simulink model "DC_Motor_Load"  (R2015a)
settings: Solver=ode45  StartTime=0.0  StopTime=10.0  RelTol=1e-3
values from neighbouring files (symbols this model uses):
  BL = B_roller + B_material    (= 0)    [dc_motor_show_data_last.m]    (also in dc_motor_show_data_last_pos.m)
  Bm = 0.0158    [dc_motor_show_data_last.m]    (also in dc_motor_show_data_last_pos.m = 0.00093)
  JL = J_roller + J_material    (= 0.000102958)    [dc_motor_show_data_last.m]    (also in dc_motor_show_data_last_pos.m)
  Jm = 0.00252    [dc_motor_show_data_last.m]    (also in dc_motor_show_data_last_pos.m = 5.26e-05)
  Kd = Kp*Td    (= 8.33268608414)    [ZIEGLER_NICHOLCUS_METHOD_tuning_pid.m]    (also in dc_motor_show_data.m = 0.0189; dc_motor_show_data_PID_range_errors_show.m = 0.09; dc_motor_show_data_PID_range_response.m = 0.09; dc_motor_show_data_PID_test_ST.m = 0.09)
  Ke = 0.1    [DC_MOTOR.m]    (also in ZIEGLER_NICHOLCUS_METHOD_tuning_pid.m = 0.57; dc_motor_show_data.m = 0.57; dc_motor_show_data_PID_range_errors_show.m; dc_motor_show_data_PID_range_response.m)
  Ki = Kp/Ti    (= 21.5184713376)    [ZIEGLER_NICHOLCUS_METHOD_tuning_pid.m]    (also in dc_motor_show_data.m = 39.9; dc_motor_show_data_PID_range_errors_show.m = 2.98; dc_motor_show_data_PID_range_response.m = 2.98; dc_motor_show_data_PID_test_ST.m = 2.98)
  Kp = 0.2*K_cr    (= 16.4)    [ZIEGLER_NICHOLCUS_METHOD_tuning_pid.m]    (also in dc_motor_show_data.m = 2.1398; dc_motor_show_data_PID_range_errors_show.m = 1.25; dc_motor_show_data_PID_range_response.m = 1.25; dc_motor_show_data_PID_test_ST.m = 1.25)
  Kt = 0.2    [DC_MOTOR.m]    (also in ZIEGLER_NICHOLCUS_METHOD_tuning_pid.m = 0.259; dc_motor_show_data.m = 0.259; dc_motor_show_data_PID_range_errors_show.m; dc_motor_show_data_PID_range_response.m)
  La = 0.143    [dc_motor_show_data_last.m]    (also in dc_motor_show_data_last_pos.m = 0.0006)
  Ra = 9.375    [dc_motor_show_data_last.m]    (also in dc_motor_show_data_last_pos.m)
  TL = 0.0017    [dc_motor_show_data_last.m]    (also in dc_motor_show_data_last_pos.m)
libraries: simulink x1
settings Model: Creator=Alfa maSR  LastModifiedBy=Alfa maSR

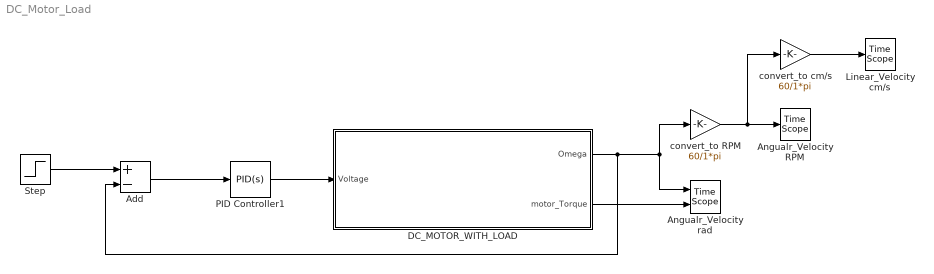
== system DC_Motor_Load ==
  Add : Sum  Inputs=+-
  Angualr_Velocity RPM : TimeScope  DefaultConfigurationName=spbscopes.TimeScopeBlockCfg
  Angualr_Velocity rad : TimeScope  DefaultConfigurationName=spbscopes.TimeScopeBlockCfg  NumInputPorts=2
  DC_MOTOR_WITH_LOAD : Subsystem
  Linear_Velocity cm/s : TimeScope  DefaultConfigurationName=spbscopes.TimeScopeBlockCfg
  PID Controller1 : simulink/Continuous/PID Controller  Controller=PID  TimeDomain=Continuous-time  SampleTime=-1  IntegratorMethod=Forward Euler  FilterMethod=Forward Euler  Form=Parallel  UseFilter=on  ControllerParametersSource=internal  P=Kp  I=Ki  D=Kd  N=100  InitialConditionSource=internal  InitialConditionForIntegrator=0  InitialConditionForFilter=0  ExternalReset=none  LimitOutput=off  UpperSaturationLimit=inf  LowerSaturationLimit=-inf  LinearizeAsGain=on  AntiWindupMode=none  Kb=1  TrackingMode=off  Kt=1  PParamMin=[]  PParamMax=[]  IParamMin=[]  IParamMax=[]  DParamMin=[]  DParamMax=[]  NParamMin=[]  NParamMax=[]  KbParamMin=[]  KbParamMax=[]  KtParamMin=[]  KtParamMax=[]  POutMin=[]  POutMax=[]  IOutMin=[]  IOutMax=[]  DOutMin=[]  DOutMax=[]  NOutMin=[]  NOutMax=[]  KbOutMin=[]  KbOutMax=[]  KtOutMin=[]  KtOutMax=[]  IntegratorOutMin=[]  IntegratorOutMax=[]  FilterOutMin=[]  FilterOutMax=[]  SumOutMin=[]  SumOutMax=[]  SumI1OutMin=[]  SumI1OutMax=[]  SumI2OutMin=[]  SumI2OutMax=[]  SumI3OutMin=[]  SumI3OutMax=[]  SumDOutMin=[]  SumDOutMax=[]  SaturationOutMin=[]  SaturationOutMax=[]  IntegratorContinuousStateAttributes=''  IntegratorStateMustResolveToSignalObject=off  IntegratorRTWStateStorageClass=Auto  FilterContinuousStateAttributes=''  FilterStateMustResolveToSignalObject=off  FilterRTWStateStorageClass=Auto  DifferentiatorICPrevScaledInput=0  DifferentiatorOutMin=[]  DifferentiatorOutMax=[]
  Step : Step  Time=0  SampleTime=0
  convert_to RPM : Gain  Gain=60/1*pi
  convert_to cm/s : Gain  Gain=60/1*pi
  wires:
  convert_to RPM/1 -> Angualr_Velocity RPM/1, convert_to cm/s/1
  convert_to cm/s/1 -> Linear_Velocity cm/s/1
  DC_MOTOR_WITH_LOAD/1(Omega) -> Add/2, convert_to RPM/1, Angualr_Velocity rad/1
  DC_MOTOR_WITH_LOAD/2(motor_Torque) -> Angualr_Velocity rad/2
  PID Controller1/1 -> DC_MOTOR_WITH_LOAD/1(Voltage)
  Add/1 -> PID Controller1/1
  Step/1 -> Add/1

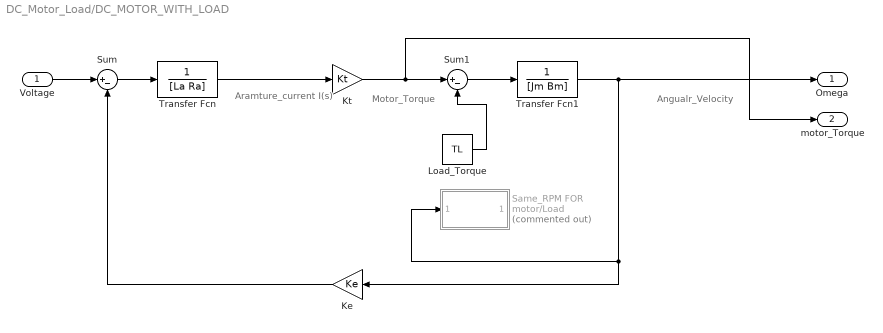
== system DC_Motor_Load/DC_MOTOR_WITH_LOAD ==
  note: Angualr_Velocity
  note: Motor_Torque
  note: Aramture_current
      |           I(s)
  Voltage : Inport
  Ke : Gain  Gain=Ke
  Kt : Gain  Gain=Kt
  Load_Torque : Constant  Value=TL
  Same_RPM FOR motor/Load : Subsystem  Commented=on
  Sum : Sum  Inputs=|+-
  Sum1 : Sum  Inputs=|+-
  Transfer Fcn : TransferFcn  Denominator=[La Ra]
  Transfer Fcn1 : TransferFcn  Denominator=[Jm Bm]
  Omega : Outport
  motor_Torque : Outport  Port=2
  wires:
  Ke/1 -> Sum/2
  Sum1/1 -> Transfer Fcn1/1
  Load_Torque/1 -> Sum1/2
  Sum/1 -> Transfer Fcn/1
  Transfer Fcn/1 -> Kt/1
  Kt/1 -> motor_Torque/1, Sum1/1
  Transfer Fcn1/1 -> Omega/1, Ke/1, Same_RPM FOR motor/Load/1(Omega/ rad/s)
  Voltage/1 -> Sum/1

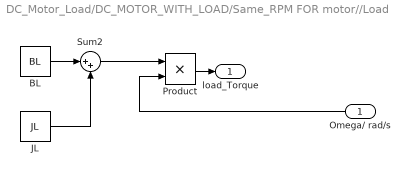
== system DC_Motor_Load/DC_MOTOR_WITH_LOAD/Same_RPM FOR motor//Load ==
  Omega/ rad/s : Inport
  BL : Constant  Value=BL
  JL : Constant  Value=JL
  Product : Product
  Sum2 : Sum  Inputs=|++
  load_Torque : Outport
  wires:
  JL/1 -> Sum2/2
  Omega/ rad/s/1 -> Product/2
  Product/1 -> load_Torque/1
  BL/1 -> Sum2/1
  Sum2/1 -> Product/1
